simulink model "CCCV_v4"  (R2019a)
settings: Solver=FixedStepAuto  StartTime=0.0  StopTime=10000  FixedStep=1  RelTol=1e-3
undefined symbols (not defined in the file or in its folder): x0_nom
libraries: simulink x1
settings Model: Creator=ztakeo  LastModifiedBy=zgima

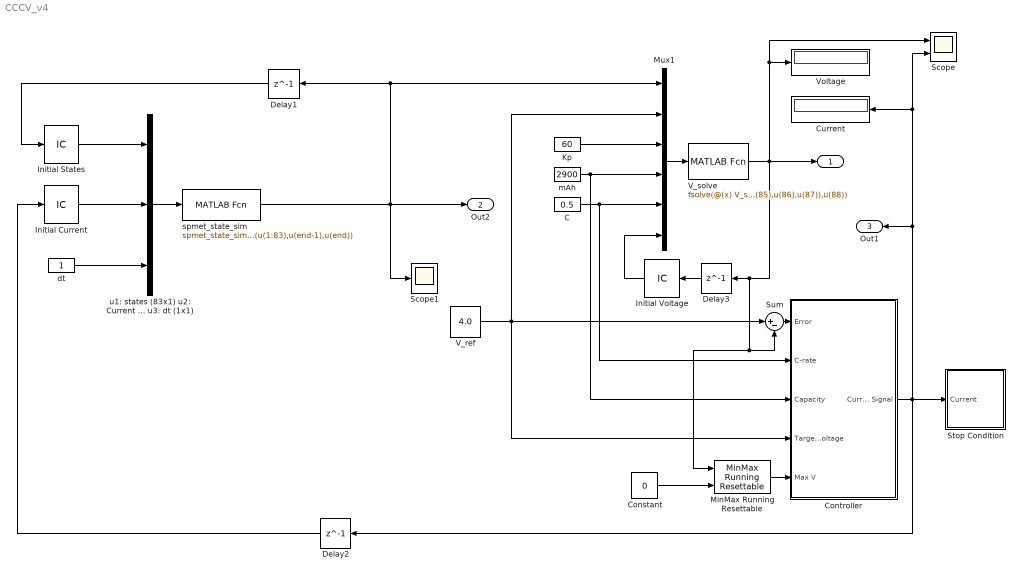
== system CCCV_v4 ==
  C : Constant  Value=0.5
  Constant : Constant  Value=0
  Controller : Subsystem
  Current : Display
  Delay1 : Delay  DelayLength=1  InitialCondition=0
  Delay2 : Delay  DelayLength=1  InitialCondition=0
  Delay3 : Delay  DelayLength=1  InitialCondition=0
  Initial Current : InitialCondition  Value=0
  "Initial States " : InitialCondition  Value=x0_nom
  "Initial Voltage " : InitialCondition  Value=2.8
  Kp : Constant  Value=60
  MinMax Running Resettable : simulink/Math Operations/MinMax Running Resettable  Function=max  vinit=0.0
  Mux1 : Mux  Inputs=6
  Scope : Scope  NumInputPorts=2
  Scope1 : Scope
  Stop Condition : Subsystem
  Sum : Sum  Inputs=|+-
  "V_ref " : Constant  Value=4.0
  V_solve : MATLABFcn  MATLABFcn=fsolve(@(x) V_solve(x, u(1:83), u(84),u(85),u(86),u(87)),u(88))  OutputDimensions=1
  "Voltage " : Display
  dt : Constant
  mAh : Constant  Value=2900
  spmet_state_sim : MATLABFcn  MATLABFcn=spmet_state_sim(u(1:83),u(end-1),u(end))  OutputDimensions=83  OutputSignalType=real
  "u1: states (83x1) u2: Current (1x1) u3: dt (1x1) " : Mux  Inputs=3
  " " : Outport  SignalName=V
  Out2 : Outport  Port=2  SignalName=x
  Out1 : Outport  Port=3  SignalName=Current
  wires:
  spmet_state_sim/1 -> Mux1/1, Delay1/1, Out2/1, Scope1/1
  Delay3/1 -> "Initial Voltage "/1
  Delay1/1 -> "Initial States "/1
  Controller/1(Current Signal) -> Scope/2, Current/1, Out1/1, Delay2/1, Stop Condition/1(Current)
  Mux1/1 -> V_solve/1
  Initial Current/1 -> "u1: states (83x1) u2: Current (1x1) u3: dt (1x1) "/2
  "V_ref "/1 -> Controller/4(Target Voltage), Sum/1, Mux1/2
  mAh/1 -> Controller/3(Capacity), Mux1/4
  Delay2/1 -> Initial Current/1
  "u1: states (83x1) u2: Current (1x1) u3: dt (1x1) "/1 -> spmet_state_sim/1
  C/1 -> Mux1/5, Controller/2(C-rate)
  "Initial States "/1 -> "u1: states (83x1) u2: Current (1x1) u3: dt (1x1) "/1
  "Initial Voltage "/1 -> Mux1/6
  Kp/1 -> Mux1/3
  dt/1 -> "u1: states (83x1) u2: Current (1x1) u3: dt (1x1) "/3
  V_solve/1 -> Delay3/1, MinMax Running Resettable/1, Sum/2, " "/1, Scope/1, "Voltage "/1
  Constant/1 -> MinMax Running Resettable/2
  MinMax Running Resettable/1 -> Controller/5(Max V)
  Sum/1 -> Controller/1(Error)

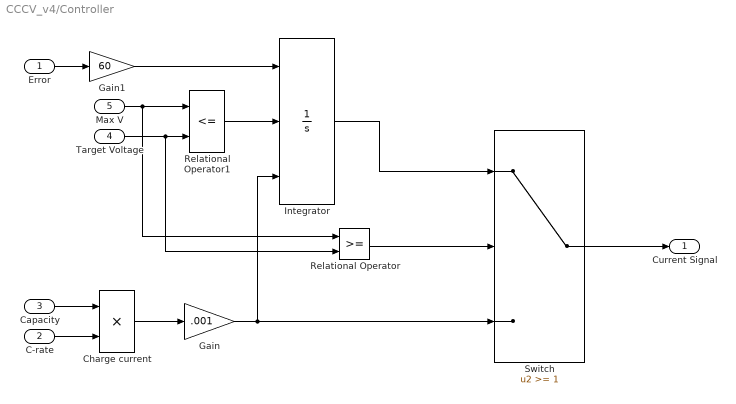
== system CCCV_v4/Controller ==
  Error : Inport
  C-rate : Inport  Port=2
  Capacity : Inport  Port=3
  Target Voltage : Inport  Port=4
  Max V : Inport  Port=5
  Charge current : Product
  Gain : Gain  Gain=.001
  Gain1 : Gain  Gain=60
  Integrator : Integrator  ExternalReset=level  InitialConditionSource=external
  Relational Operator : RelationalOperator  OutDataTypeStr=boolean  RndMeth=Nearest
  Relational Operator1 : RelationalOperator  Operator=<=  OutDataTypeStr=boolean  RndMeth=Nearest
  Switch : Switch  Threshold=1
  Current Signal : Outport
  wires:
  Error/1 -> Gain1/1
  Target Voltage/1 -> Relational Operator/2, Relational Operator1/2
  Switch/1 -> Current Signal/1
  C-rate/1 -> Charge current/2
  Capacity/1 -> Charge current/1
  Gain/1 -> Switch/3, Integrator/3
  Relational Operator1/1 -> Integrator/2
  Max V/1 -> Relational Operator/1, Relational Operator1/1
  Gain1/1 -> Integrator/1
  Charge current/1 -> Gain/1
  Integrator/1 -> Switch/1
  Relational Operator/1 -> Switch/2

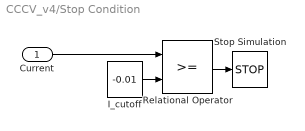
== system CCCV_v4/Stop Condition ==
  Current : Inport
  I_cutoff : Constant  Value=-0.01
  Relational Operator : RelationalOperator  OutDataTypeStr=boolean  RndMeth=Simplest
  Stop Simulation : Stop
  wires:
  Current/1 -> Relational Operator/1
  Relational Operator/1 -> Stop Simulation/1
  I_cutoff/1 -> Relational Operator/2
